simulink model "EPD629_WilliamsJ_AS03_simulink"  (R2021b)
settings: Solver=VariableStepAuto  StartTime=0.0  StopTime=2000  RelTol=1e-3
values from neighbouring files (symbols this model uses):
  AeroArea_m2 = 10    [EPD629_WilliamsJ_AS03_SimulinkScript.m.m]
  AeroDragCoef = 0.6    [EPD629_WilliamsJ_AS03_SimulinkScript.m.m]
  AirGasConstant_kJpkgK = 0.278    [EPD629_WilliamsJ_AS03_SimulinkScript.m.m]
  AmbientPress_kPa = 100    [EPD629_WilliamsJ_AS03_SimulinkScript.m.m]
  AmbientTemp_C = 20    [EPD629_WilliamsJ_AS03_SimulinkScript.m.m]
  AxleRatio = 3.25    [EPD629_WilliamsJ_AS03_SimulinkScript.m.m]
  CelsiusToKelvinConstant = 273.15    [EPD629_WilliamsJ_AS03_SimulinkScript.m.m]
  EngineFrictionData_Nm = C(1) + C(2) * EngineSpeedBreakpoints_rpm + C(3) * EngineSpeedBreakpoints_rpm .^2    [EPD629_WilliamsJ_AS03_SimulinkScript.m.m]
  EngineSpeedBreakpoints_rpm = [900, 1000, 1100, 1160, 1200, 1300, 1400, 1500, 1600, 1700, 1800, 1900, 2000]    [EPD629_WilliamsJ_AS03_SimulinkScript.m.m]
  EngineTorqueMaxData_Nm = EngineTorqueMaxData_ftlb * ConversionFactor_Nm_per_ftlb    [EPD629_WilliamsJ_AS03_SimulinkScript.m.m]
  EngineTorqueTimeConstant_s = 0.1    [EPD629_WilliamsJ_AS03_SimulinkScript.m.m]
  GravitationalAccel_mps2 = 9.8067    [EPD629_WilliamsJ_AS03_SimulinkScript.m.m]
  PitchAngleData_deg = [2 2]    [EPD629_WilliamsJ_AS03_SimulinkScript.m.m]
  PitchAnglePositionBP_m = [0 1e6]    [EPD629_WilliamsJ_AS03_SimulinkScript.m.m]
  RollingDragCoef = 0.005    [EPD629_WilliamsJ_AS03_SimulinkScript.m.m]
  TireRevsPerKilometer = TireRevsPerMile * ConversionFactor_mile_per_km    (= 310.6855)    [EPD629_WilliamsJ_AS03_SimulinkScript.m.m]
  TransGearRatioData = [14.43, 11.05, 8.44, 6.46, 4.95, 3.79, 2.91, 2.23, 1.70, 1.30, 1.00, 0.77]    [EPD629_WilliamsJ_AS03_SimulinkScript.m.m]
  VehicleMass_kg = 30000    [EPD629_WilliamsJ_AS03_SimulinkScript.m.m]
settings Model: Creator=jwilli42  LastModifiedBy=Justin

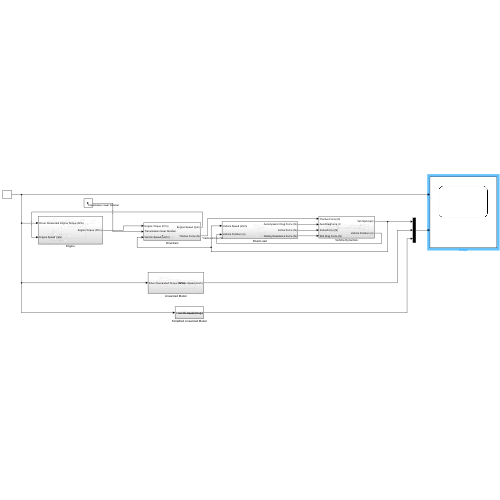
[thumbnail: Simulink's stored preview of the top-level diagram]
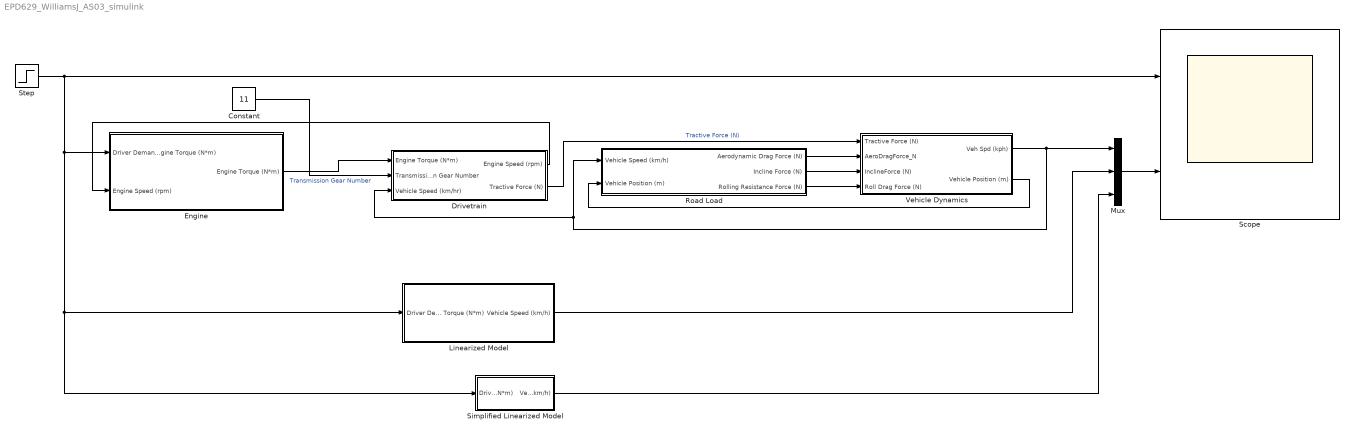
== system EPD629_WilliamsJ_AS03_simulink ==
  Constant : Constant  Value=11
  Drivetrain : Subsystem
  Engine : Subsystem
  Linearized Model : Subsystem
  Mux : Mux  Inputs=3
  Road Load : Subsystem
  Scope : Scope  NumInputPorts=2
  Simplified Linearized Model : Subsystem
  Step : Step  Time=1000  Before=2450  After=2550  SampleTime=0
  Vehicle Dynamics : Subsystem
  wires:
  Vehicle Dynamics/1(Veh Spd (kph)) -> Mux/1, Drivetrain/3(Vehicle Speed (km/hr)), Road Load/1(Vehicle Speed (km/h))
  Vehicle Dynamics/2(Vehicle Position (m)) -> Road Load/2(Vehicle Position (m))
  Road Load/3(Rolling Resistance Force (N)) -> Vehicle Dynamics/4(Roll Drag Force (N))
  Drivetrain/2(Tractive Force (N)) -> Vehicle Dynamics/1(Tractive Force (N))  "Tractive Force (N)"
  Road Load/1(Aerodynamic Drag Force (N)) -> Vehicle Dynamics/2(AeroDragForce_N)
  Road Load/2(Incline Force (N)) -> Vehicle Dynamics/3(InclineForce (N))
  Engine/1(Engine Torque (N*m)) -> Drivetrain/1(Engine Torque (N*m))
  Drivetrain/1(Engine Speed (rpm)) -> Engine/2(Engine Speed (rpm))
  Constant/1 -> Drivetrain/2(Transmission Gear Number)  "Transmission Gear Number"
  Step/1 -> Engine/1(Driver Demanded Engine Torque (N*m)), Simplified Linearized Model/1(Driver Demanded Engine Torque (N*m)), Linearized Model/1(Driver Demanded Torque (N*m)), Scope/1
  Linearized Model/1(Vehicle Speed (km/h)) -> Mux/2
  Simplified Linearized Model/1(Vehicle Speed (km/h)) -> Mux/3
  Mux/1 -> Scope/2

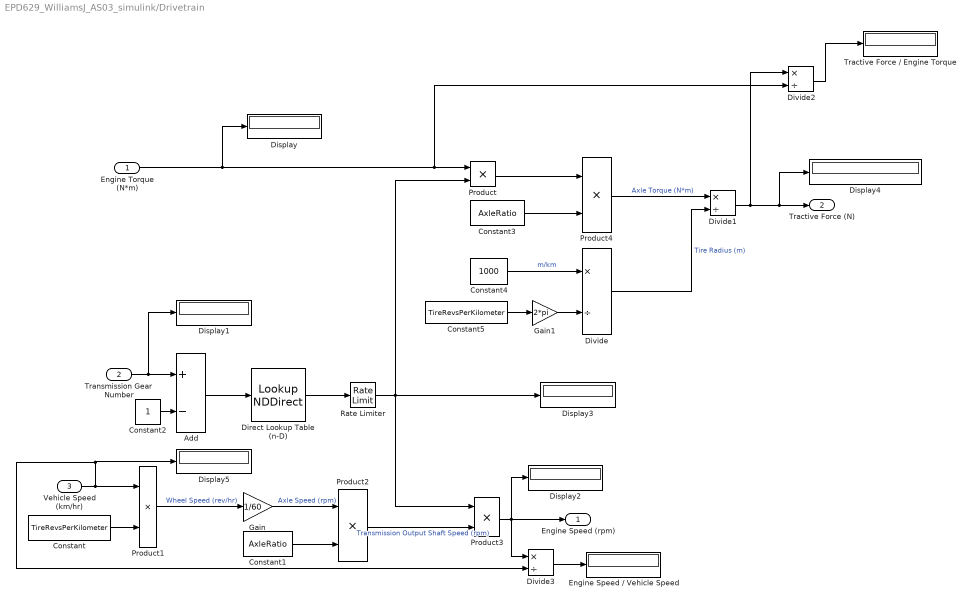
== system EPD629_WilliamsJ_AS03_simulink/Drivetrain ==
  Engine Torque (N*m) : Inport
  Transmission Gear Number : Inport  Port=2
  Vehicle Speed (km/hr) : Inport  Port=3
  Add : Sum  Inputs=+-
  Constant : Constant  Value=TireRevsPerKilometer
  Constant1 : Constant  Value=AxleRatio
  Constant2 : Constant
  Constant3 : Constant  Value=AxleRatio
  Constant4 : Constant  Value=1000
  Constant5 : Constant  Value=TireRevsPerKilometer
  Direct Lookup Table (n-D) : LookupNDDirect  NumberOfTableDimensions=1  Table=TransGearRatioData
  Display{,1..5} (6 alike) : Display
  Divide{,1..3} (4 alike) : Product  Inputs=*/
  Engine Speed / Vehicle Speed : Display
  Gain : Gain  Gain=1/60
  Gain1 : Gain  Gain=2*pi
  Product{,1..4} (5 alike) : Product
  Rate Limiter : RateLimiter  RisingSlewLimit=5  FallingSlewLimit=-5  SampleTimeMode=inherited
  Tractive Force / Engine Torque : Display
  Engine Speed (rpm) : Outport
  Tractive Force (N) : Outport  Port=2
  wires:
  Product/1 -> Product4/1
  Engine Torque (N*m)/1 -> Display/1, Divide2/2, Product/1
  Vehicle Speed (km/hr)/1 -> Divide3/2, Display5/1, Product1/1
  Constant/1 -> Product1/2
  Product1/1 -> Gain/1  "Wheel Speed (rev/hr)"
  Gain/1 -> Product2/1  "Axle Speed (rpm)"
  Constant1/1 -> Product2/2
  Product2/1 -> Product3/2  "Transmission Output Shaft Speed (rpm)"
  Transmission Gear Number/1 -> Display1/1, Add/1
  Constant2/1 -> Add/2
  Product3/1 -> Divide3/1, Display2/1, Engine Speed (rpm)/1
  Constant3/1 -> Product4/2
  Constant4/1 -> Divide/1  "m/km"
  Constant5/1 -> Gain1/1
  Gain1/1 -> Divide/2
  Product4/1 -> Divide1/1  "Axle Torque (N*m)"
  Divide/1 -> Divide1/2  "Tire Radius (m)"
  Divide1/1 -> Divide2/1, Display4/1, Tractive Force (N)/1
  Rate Limiter/1 -> Product/2, Display3/1, Product3/1
  Direct Lookup Table (n-D)/1 -> Rate Limiter/1
  Add/1 -> Direct Lookup Table (n-D)/1
  Divide2/1 -> Tractive Force / Engine Torque/1
  Divide3/1 -> Engine Speed / Vehicle Speed/1

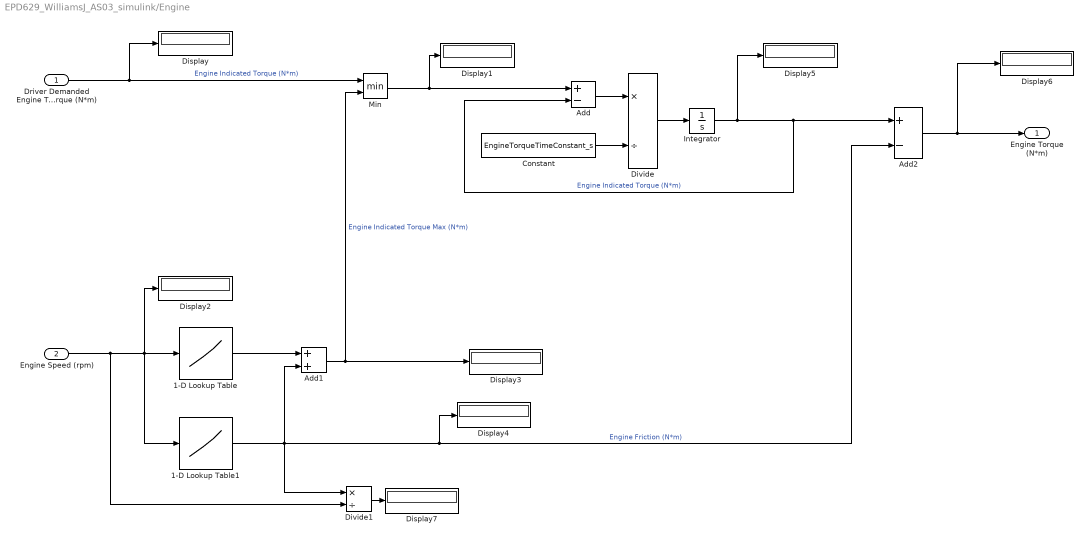
== system EPD629_WilliamsJ_AS03_simulink/Engine ==
  Driver Demanded Engine Torque (N*m) : Inport
  Engine Speed (rpm) : Inport  Port=2
  1-D Lookup Table : Lookup_n-D  NumberOfTableDimensions=1  BreakpointsForDimension1=EngineSpeedBreakpoints_rpm  Table=EngineTorqueMaxData_Nm  ExtrapMethod=Clip  UseLastTableValue=on  InternalRulePriority=Speed  RndMeth=Simplest  InputSameDT=on
  1-D Lookup Table1 : Lookup_n-D  NumberOfTableDimensions=1  BreakpointsForDimension1=EngineSpeedBreakpoints_rpm  Table=EngineFrictionData_Nm  ExtrapMethod=Clip  UseLastTableValue=on  InternalRulePriority=Speed  RndMeth=Simplest  InputSameDT=on
  Add : Sum  Inputs=+-
  Add1 : Sum
  Add2 : Sum  Inputs=+-
  Constant : Constant  Value=EngineTorqueTimeConstant_s
  Display{,1..7} (8 alike) : Display
  Divide : Product  Inputs=*/
  Divide1 : Product  Inputs=*/
  Integrator : Integrator  InitialCondition=2494.7  LimitOutput=on  UpperSaturationLimit=3000  LowerSaturationLimit=0
  Min : MinMax  Inputs=2
  Engine Torque (N*m) : Outport
  wires:
  Driver Demanded Engine Torque (N*m)/1 -> Min/1, Display/1  "Engine Indicated Torque (N*m)"
  1-D Lookup Table/1 -> Add1/1
  Engine Speed (rpm)/1 -> Divide1/2, 1-D Lookup Table/1, Display2/1, 1-D Lookup Table1/1
  Min/1 -> Display1/1, Add/1
  Add1/1 -> Display3/1, Min/2  "Engine Indicated Torque Max (N*m)"
  Add/1 -> Divide/1
  1-D Lookup Table1/1 -> Divide1/1, Add1/2, Display4/1, Add2/2  "Engine Friction (N*m)"
  Divide/1 -> Integrator/1
  Integrator/1 -> Display5/1, Add2/1, Add/2  "Engine Indicated Torque (N*m)"
  Add2/1 -> Display6/1, Engine Torque (N*m)/1
  Constant/1 -> Divide/2
  Divide1/1 -> Display7/1

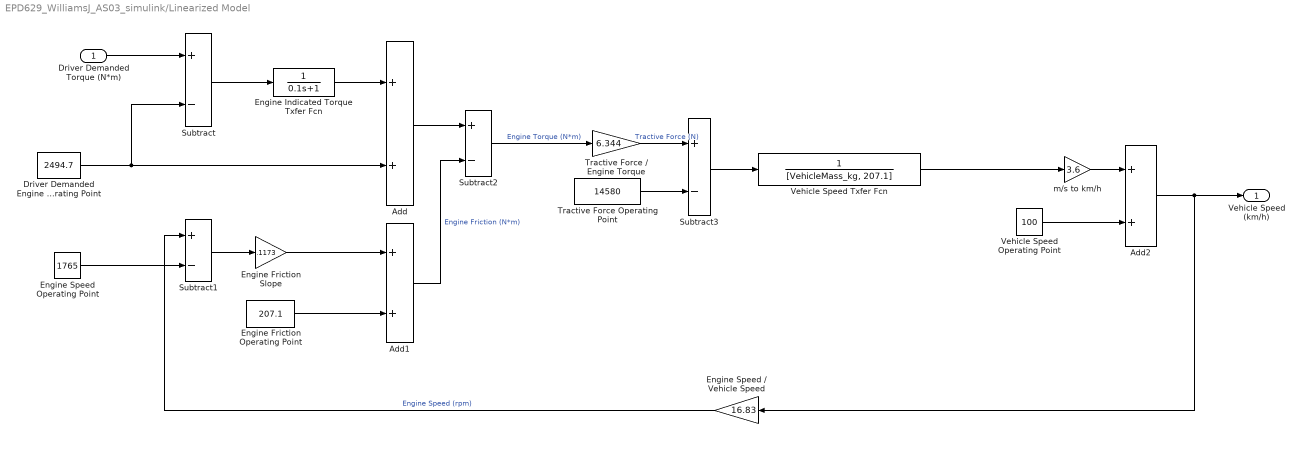
== system EPD629_WilliamsJ_AS03_simulink/Linearized Model ==
  Driver Demanded Torque (N*m) : Inport
  Add : Sum
  Add1 : Sum
  Add2 : Sum
  Driver Demanded Engine Torque Operating Point : Constant  Value=2494.7
  Engine Friction Operating Point : Constant  Value=207.1
  Engine Friction Slope : Gain  Gain=.1173
  Engine Indicated Torque Txfer Fcn : TransferFcn  Denominator=[0.1 1]
  Engine Speed / Vehicle Speed : Gain  Gain=16.83
  Engine Speed Operating Point : Constant  Value=1765
  Subtract{,1..3} (4 alike) : Sum  Inputs=+-
  Tractive Force / Engine Torque : Gain  Gain=6.344
  Tractive Force Operating Point : Constant  Value=14580
  Vehicle Speed Operating Point : Constant  Value=100
  Vehicle Speed Txfer Fcn : TransferFcn  Denominator=[VehicleMass_kg, 207.1]
  m/s to km/h : Gain  Gain=3.6
  Vehicle Speed (km/h) : Outport
  wires:
  Driver Demanded Torque (N*m)/1 -> Subtract/1
  Driver Demanded Engine Torque Operating Point/1 -> Subtract/2, Add/2
  Subtract/1 -> Engine Indicated Torque Txfer Fcn/1
  Engine Indicated Torque Txfer Fcn/1 -> Add/1
  Subtract1/1 -> Engine Friction Slope/1
  Engine Friction Slope/1 -> Add1/1
  Engine Friction Operating Point/1 -> Add1/2
  Add/1 -> Subtract2/1
  Add1/1 -> Subtract2/2  "Engine Friction (N*m)"
  Subtract2/1 -> Tractive Force / Engine Torque/1  "Engine Torque (N*m)"
  Tractive Force Operating Point/1 -> Subtract3/2
  Subtract3/1 -> Vehicle Speed Txfer Fcn/1
  Vehicle Speed Txfer Fcn/1 -> m/s to km/h/1
  m/s to km/h/1 -> Add2/1
  Add2/1 -> Engine Speed / Vehicle Speed/1, Vehicle Speed (km/h)/1
  Engine Speed / Vehicle Speed/1 -> Subtract1/1  "Engine Speed (rpm)"
  Vehicle Speed Operating Point/1 -> Add2/2
  Tractive Force / Engine Torque/1 -> Subtract3/1  "Tractive Force (N)"
  Engine Speed Operating Point/1 -> Subtract1/2

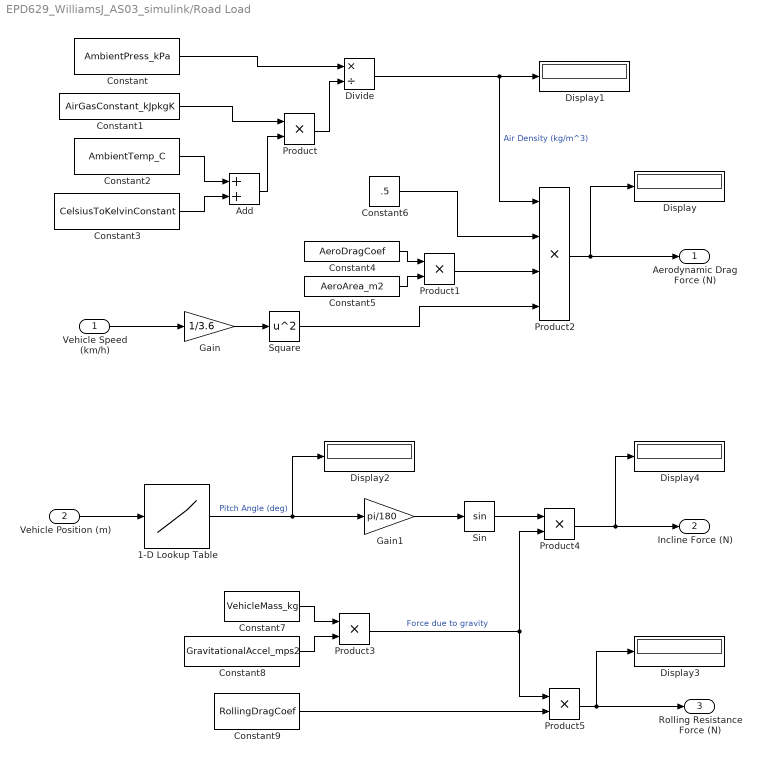
== system EPD629_WilliamsJ_AS03_simulink/Road Load ==
  Vehicle Speed (km/h) : Inport
  Vehicle Position (m) : Inport  Port=2
  1-D Lookup Table : Lookup_n-D  NumberOfTableDimensions=1  BreakpointsForDimension1=PitchAnglePositionBP_m  Table=PitchAngleData_deg  ExtrapMethod=Clip  UseLastTableValue=on  InternalRulePriority=Speed  RndMeth=Simplest  InputSameDT=on
  Add : Sum
  Constant : Constant  Value=AmbientPress_kPa
  Constant1 : Constant  Value=AirGasConstant_kJpkgK
  Constant2 : Constant  Value=AmbientTemp_C
  Constant3 : Constant  Value=CelsiusToKelvinConstant
  Constant4 : Constant  Value=AeroDragCoef
  Constant5 : Constant  Value=AeroArea_m2
  Constant6 : Constant  Value=.5
  Constant7 : Constant  Value=VehicleMass_kg
  Constant8 : Constant  Value=GravitationalAccel_mps2
  Constant9 : Constant  Value=RollingDragCoef
  Display{,1..4} (5 alike) : Display
  Divide : Product  Inputs=*/
  Gain : Gain  Gain=1/3.6
  Gain1 : Gain  Gain=pi/180
  Product{,1,3..5} (5 alike) : Product
  Product2 : Product  Inputs=4
  Sin : Trigonometry
  Square : Math  Operator=square  SaturateOnIntegerOverflow=on
  Aerodynamic Drag Force (N) : Outport
  Incline Force (N) : Outport  Port=2
  Rolling Resistance Force (N) : Outport  Port=3
  wires:
  Product4/1 -> Incline Force (N)/1, Display4/1
  Constant/1 -> Divide/1
  Gain1/1 -> Sin/1
  Product2/1 -> Display/1, Aerodynamic Drag Force (N)/1
  Constant3/1 -> Add/2
  Product5/1 -> Rolling Resistance Force (N)/1, Display3/1
  Constant2/1 -> Add/1
  Product3/1 -> Product5/1, Product4/2  "Force due to gravity"
  Constant7/1 -> Product3/1
  Gain/1 -> Square/1
  Divide/1 -> Product2/1, Display1/1  "Air Density (kg/m^3)"
  1-D Lookup Table/1 -> Display2/1, Gain1/1  "Pitch Angle (deg)"
  Vehicle Position (m)/1 -> 1-D Lookup Table/1
  Product/1 -> Divide/2
  Constant1/1 -> Product/1
  Add/1 -> Product/2
  Constant4/1 -> Product1/1
  Constant5/1 -> Product1/2
  Vehicle Speed (km/h)/1 -> Gain/1
  Constant6/1 -> Product2/2
  Constant8/1 -> Product3/2
  Constant9/1 -> Product5/2
  Sin/1 -> Product4/1
  Product1/1 -> Product2/3
  Square/1 -> Product2/4

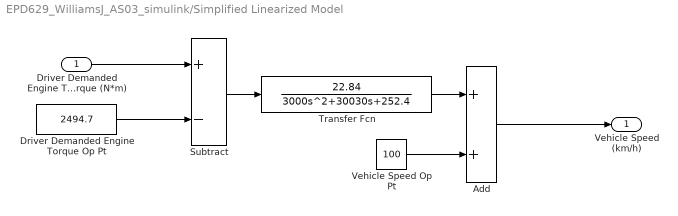
== system EPD629_WilliamsJ_AS03_simulink/Simplified Linearized Model ==
  Driver Demanded Engine Torque (N*m) : Inport
  Add : Sum
  Driver Demanded Engine Torque Op Pt : Constant  Value=2494.7
  Subtract : Sum  Inputs=+-
  Transfer Fcn : TransferFcn  Numerator=[22.84]  Denominator=[3000, 30030, 252.4]
  Vehicle Speed Op Pt : Constant  Value=100
  Vehicle Speed (km/h) : Outport
  wires:
  Driver Demanded Engine Torque (N*m)/1 -> Subtract/1
  Driver Demanded Engine Torque Op Pt/1 -> Subtract/2
  Subtract/1 -> Transfer Fcn/1
  Transfer Fcn/1 -> Add/1
  Vehicle Speed Op Pt/1 -> Add/2
  Add/1 -> Vehicle Speed (km/h)/1

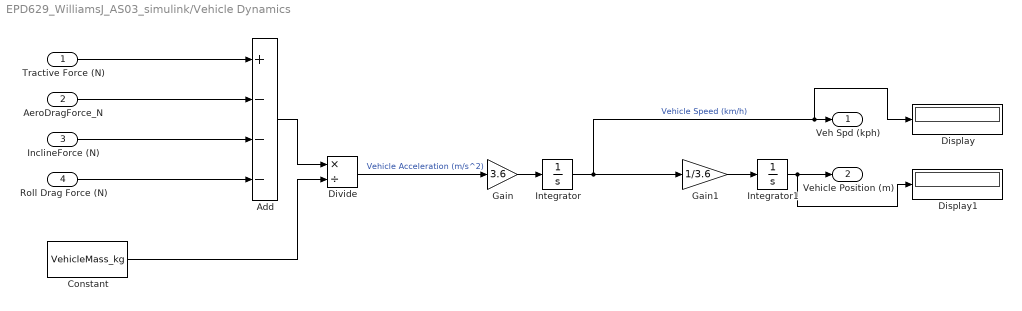
== system EPD629_WilliamsJ_AS03_simulink/Vehicle Dynamics ==
  Tractive Force (N) : Inport
  AeroDragForce_N : Inport  Port=2
  InclineForce (N) : Inport  Port=3
  Roll Drag Force (N) : Inport  Port=4
  Add : Sum  Inputs=+---
  Constant : Constant  Value=VehicleMass_kg
  Display : Display
  Display1 : Display
  Divide : Product  Inputs=*/
  Gain : Gain  Gain=3.6
  Gain1 : Gain  Gain=1/3.6
  Integrator : Integrator  InitialCondition=100  LimitOutput=on  UpperSaturationLimit=150  LowerSaturationLimit=0
  Integrator1 : Integrator  LimitOutput=on  UpperSaturationLimit=1e6  LowerSaturationLimit=0
  Veh Spd (kph) : Outport
  Vehicle Position (m) : Outport  Port=2
  wires:
  Gain/1 -> Integrator/1
  AeroDragForce_N/1 -> Add/2
  Roll Drag Force (N)/1 -> Add/4
  Integrator1/1 -> Vehicle Position (m)/1, Display1/1
  Divide/1 -> Gain/1  "Vehicle Acceleration (m/s^2)"
  InclineForce (N)/1 -> Add/3
  Integrator/1 -> Display/1, Veh Spd (kph)/1, Gain1/1  "Vehicle Speed (km/h)"
  Gain1/1 -> Integrator1/1
  Constant/1 -> Divide/2
  Tractive Force (N)/1 -> Add/1
  Add/1 -> Divide/1
